simulink model "simMinTimeTraj"  (R2016b)
settings: Solver=ode4  StartTime=0.0  StopTime=tf_  FixedStep=0.01  RelTol=1e-3
undefined symbols (not defined in the file or in its folder): apiece, tpiece, v0_, x0_
settings Model: Creator=ssk  LastModifiedBy=ssk

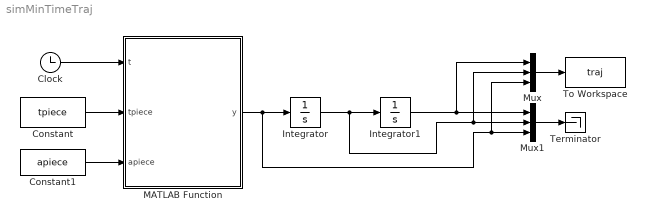
== system simMinTimeTraj ==
  Clock : Clock
  Constant : Constant  Value=tpiece
  Constant1 : Constant  Value=apiece
  Integrator : Integrator  InitialCondition=v0_
  Integrator1 : Integrator  InitialCondition=x0_
  MATLAB Function : MATLAB Function  TreatAsAtomicUnit=on
  Mux : Mux  Inputs=3
  Mux1 : Mux  Inputs=3
  Terminator : Terminator
  To Workspace : ToWorkspace  VariableName=traj  SaveFormat=Timeseries  SampleTime=-1
  wires:
  Clock/1 -> MATLAB Function/1(t)
  Constant/1 -> MATLAB Function/2(tpiece)
  Constant1/1 -> MATLAB Function/3(apiece)
  MATLAB Function/1(y) -> Mux1/3, Mux/3, Integrator/1
  Integrator/1 -> Mux1/2, Mux/2, Integrator1/1
  Integrator1/1 -> Mux1/1, Mux/1
  Mux/1 -> To Workspace/1
  Mux1/1 -> Terminator/1

== matlab function simMinTimeTraj/MATLAB Function ==
  data: t input; y output; tpiece input; apiece input
function y = fcn(t,tpiece,apiece)

for k=2:length(tpiece)
    if and(t <= tpiece(k), t >= tpiece(k-1))
        t01 = tpiece(k) - tpiece(k-1);
        t0t = t - tpiece(k-1);
        u = apiece(k-1) + (apiece(k) - apiece(k-1))*t0t/t01;
        break;
    else
        u = 0;
    end
end

y = u;

end
